simulink model "must_init_outputs_in_for_loops"  (Simulink 10.0)
settings: Solver=ode45  StartTime=0.0  StopTime=10.0  RelTol=1e-3  EnableMultiTasking=on
settings Model: Creator=Kerry Schutz  LastModifiedBy=bhisma
settings DataIOCC: LimitDataPoints=on  SignalLoggingSaveFormat=ModelDataLogs
settings OptimizationCC: ExpressionDepthLimit=2147483647  InitFltsAndDblsToZero=on
settings DebuggingCC: SolverPrmCheckMsg=warning  FcnCallInpInsideContextMsg=warning  StateNameClashWarn=warning
settings SFSimCC: SimUseLocalCustomCode=on  SimParseCustomCode=off  CustomCodeUndefinedFunction=FilterOut
settings RTWCC: RTWUseLocalCustomCode=on

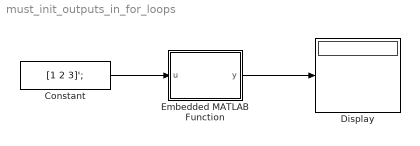
== system must_init_outputs_in_for_loops ==
  Constant : Constant  Value=[1 2 3]';  SampleTime=1
  Display : Display
  Embedded MATLAB Function : MATLAB Function  TreatAsAtomicUnit=on
  wires:
  Constant/1 -> Embedded MATLAB Function/1(u)
  Embedded MATLAB Function/1(y) -> Display/1

== matlab function Embedded MATLAB Function ==
  data: u input double; y output double
function y = fcn(u)
% y has to be initialized or this EML function won't compile
y = zeros(3,1);
for k = 1:3
   y(k) = u(k)*2;
end
